simulink model "UAV_Controller"  (R2025b)
settings: Solver=FixedStepDiscrete  StartTime=0.0  StopTime=10.0  FixedStep=0.01  RelTol=1e-3
settings Model: Creator=leonardo-avoni  LastModifiedBy=leonardo-avoni

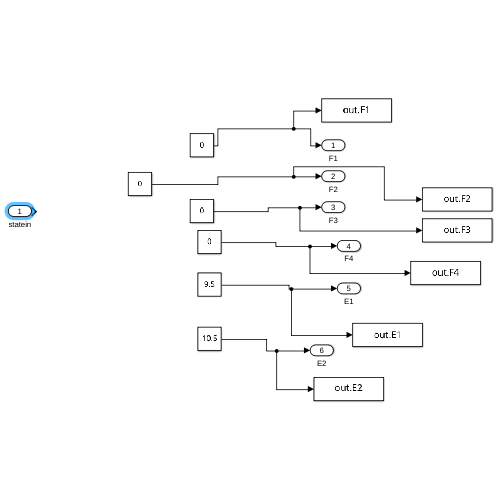
[thumbnail: Simulink's stored preview of the top-level diagram]
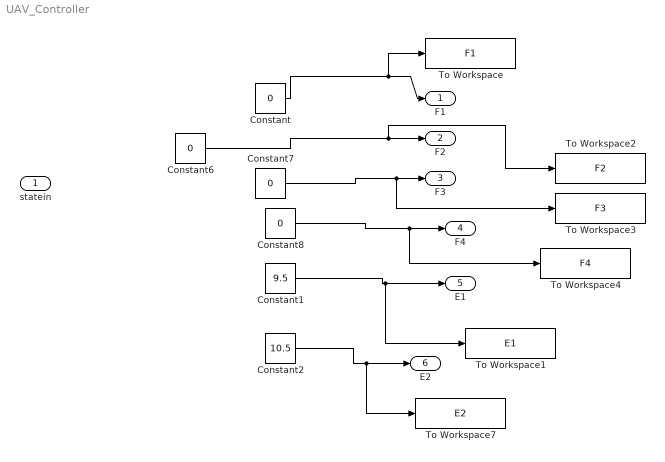
== system UAV_Controller ==
  statein : Inport  PortDimensions=1945
  Constant{,6..8} (4 alike) : Constant  Value=0
  Constant1 : Constant  Value=9.5
  Constant2 : Constant  Value=10.5
  To Workspace : ToWorkspace  VariableName=F1  SaveFormat=Timeseries  SampleTime=-1
  To Workspace1 : ToWorkspace  VariableName=E1  SaveFormat=Timeseries  SampleTime=-1
  To Workspace2 : ToWorkspace  VariableName=F2  SaveFormat=Timeseries  SampleTime=-1
  To Workspace3 : ToWorkspace  VariableName=F3  SaveFormat=Timeseries  SampleTime=-1
  To Workspace4 : ToWorkspace  VariableName=F4  SaveFormat=Timeseries  SampleTime=-1
  To Workspace7 : ToWorkspace  VariableName=E2  SaveFormat=Timeseries  SampleTime=-1
  F1 : Outport
  F2 : Outport  Port=2
  F3 : Outport  Port=3
  F4 : Outport  Port=4
  E1 : Outport  Port=5
  E2 : Outport  Port=6
  wires:
  Constant/1 -> To Workspace/1, F1/1
  Constant6/1 -> To Workspace2/1, F2/1
  Constant7/1 -> To Workspace3/1, F3/1
  Constant8/1 -> To Workspace4/1, F4/1
  Constant1/1 -> To Workspace1/1, E1/1
  Constant2/1 -> To Workspace7/1, E2/1
